simulink model "diff_controller_PID"  (R2024b)
settings: Solver=FixedStepAuto  StartTime=0.0  StopTime=inf  FixedStep=0.001  RelTol=1e-3  EnableMultiTasking=on
InitFcn:
  | Ts = 0.005;
  | diameter = 165; %mm
  | width = 441; %mm
libraries: arduinolib x4, simulink x2
settings Model: SimulationMode=external  ExtModeTrigDuration=2  Creator=System-10  LastModifiedBy=01149
settings SolverCC: AutoInsertRateTranBlk=on
settings OptimizationCC: EnhancedBackFolding=on  PassReuseOutputArgsAs=Individual arguments  ZeroExternalMemoryAtStartup=off  ZeroInternalMemoryAtStartup=off  MaxStackSize=64  OptimizeBlockOrder=speed  DifferentSizesBufferReuse=on  OptimizationCustomize=off  EfficientTunableParamExpr=on
settings DebuggingCC: ParameterTunabilityLossMsg=error
settings HardwareCC: ProdBitPerInt=16  ProdBitPerPointer=16  ProdBitPerSizeT=16  ProdBitPerPtrDiffT=16  ProdLargestAtomicFloat=None  ProdWordSize=8  ProdHWDeviceType=Atmel->AVR
settings SFSimCC: MATLABDynamicMemAlloc=off
settings RTWCC: Description=Embedded Coder  SystemTargetFile=ert.tlc  HardwareBoard=Arduino Mega 2560  TemplateMakefile=ert_default_tmf  GenerateReport=on  Toolchain=Arduino AVR  BuildConfiguration=Faster Runs  GPUComputeCapability=3.5
settings CodeAppCC: ForceParamTrailComments=on  IgnoreCustomStorageClasses=off  OperatorAnnotations=on  SimulinkDataObjDesc=on  SFDataObjDesc=on  InsertBlockDesc=on
settings ERTTargetCC: SupportContinuousTime=on  SupportVariableSizeSignals=on  ExtModeTransport=3  ExtModeStaticAlloc=on  ExtModeAutomaticAllocSize=off  ExtModeStaticAllocSize=2048  ExtModeMexFile=ext_xcp  ExtModeIntrfLevel=Level2 - Open  InlinedParameterPlacement=Hierarchical  DynamicArrayContainerType=coder::array

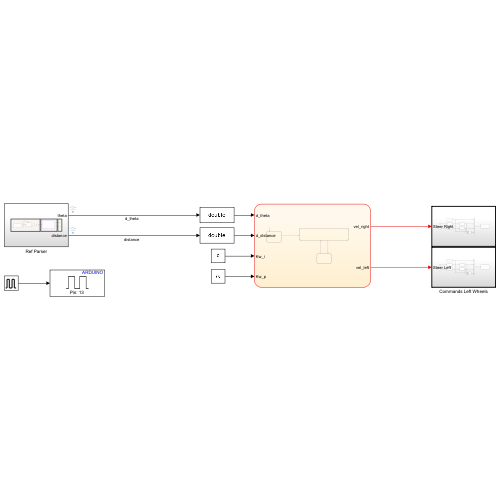
[thumbnail: Simulink's stored preview of the top-level diagram]
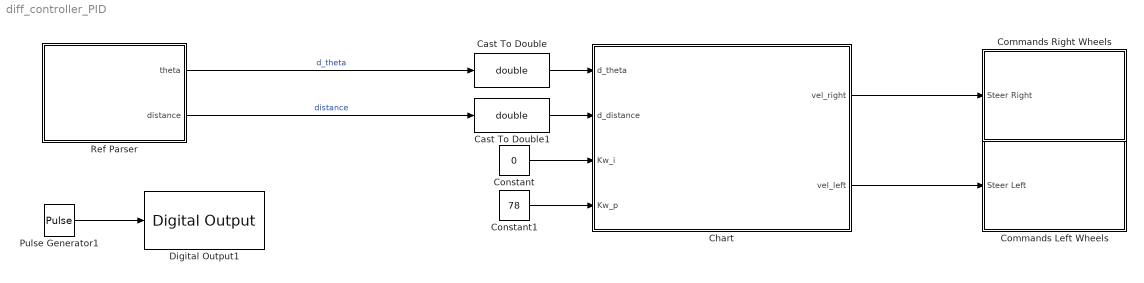
== system diff_controller_PID ==
  Cast To Double : DataTypeConversion  OutDataTypeStr=double  SaturateOnIntegerOverflow=off  RndMeth=Floor
  Cast To Double1 : DataTypeConversion  OutDataTypeStr=double  SaturateOnIntegerOverflow=off  RndMeth=Floor
  Chart : Stateflow chart  TreatAsAtomicUnit=on
  Commands Left Wheels : Subsystem  TreatAsAtomicUnit=on  SystemSampleTime=Ts
  Commands Right Wheels : Subsystem  TreatAsAtomicUnit=on  SystemSampleTime=Ts
  Constant : Constant  Value=0
  Constant1 : Constant  Value=78
  Digital Output1 : arduinolib/Digital Output  pinNumber=13  Direction=output  blockPlatform=arduino
  Pulse Generator1 : DiscretePulseGenerator  PulseType=Time based  PulseWidth=50
  Ref Parser : Subsystem
  wires:
  Pulse Generator1/1 -> Digital Output1/1
  Ref Parser/1(theta) -> Cast To Double/1  "d_theta"
  Ref Parser/2(distance) -> Cast To Double1/1  "distance"
  Constant/1 -> Chart/3(Kw_i)
  Constant1/1 -> Chart/4(Kw_p)
  Chart/1(vel_right) -> Commands Right Wheels/1(Steer Right)
  Chart/2(vel_left) -> Commands Left Wheels/1(Steer Left)
  Cast To Double/1 -> Chart/1(d_theta)
  Cast To Double1/1 -> Chart/2(d_distance)

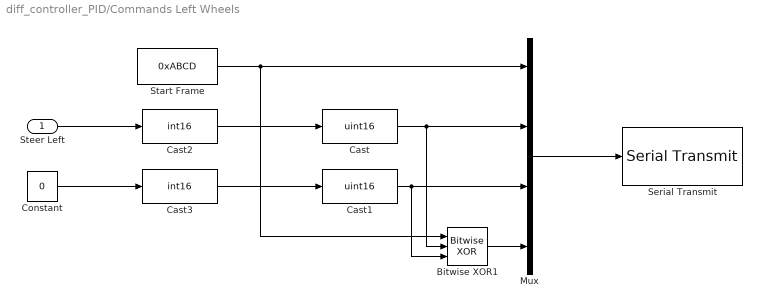
== system diff_controller_PID/Commands Left Wheels ==
  Steer Left : Inport
  Bitwise XOR1 : simulink/Logic and Bit Operations/Bitwise Operator  logicop=XOR  UseBitMask=off  NumInputPorts=3  BitMask=bin2dec('11011001')  BitMaskRealWorld=Stored Integer
      settings: LibrarySourceBlock=|
      | simulink/Quick Insert/Logic and Bit
      | Operations/Bitwise XOR
  Cast : DataTypeConversion  OutDataTypeStr=uint16  SaturateOnIntegerOverflow=off  RndMeth=Floor
  Cast1 : DataTypeConversion  OutDataTypeStr=uint16  SaturateOnIntegerOverflow=off  RndMeth=Floor
  Cast2 : DataTypeConversion  OutDataTypeStr=int16  SaturateOnIntegerOverflow=off  RndMeth=Floor
  Cast3 : DataTypeConversion  OutDataTypeStr=int16  SaturateOnIntegerOverflow=off  RndMeth=Floor
  Constant : Constant  Value=0
  Mux : Mux
  Serial Transmit : arduinolib/Serial Transmit  portNumber=3  sendmode=write  sendformat=Decimal  floatprecision=2  header=[]  terminator=[]  blockPlatform=arduino
  Start Frame : Constant  Value=0xABCD  OutDataTypeStr=uint16
  wires:
  Cast1/1 -> Bitwise XOR1/3, Mux/3
  Constant/1 -> Cast3/1
  Start Frame/1 -> Bitwise XOR1/1, Mux/1
  Mux/1 -> Serial Transmit/1
  Steer Left/1 -> Cast2/1
  Bitwise XOR1/1 -> Mux/4
  Cast/1 -> Bitwise XOR1/2, Mux/2
  Cast2/1 -> Cast/1
  Cast3/1 -> Cast1/1

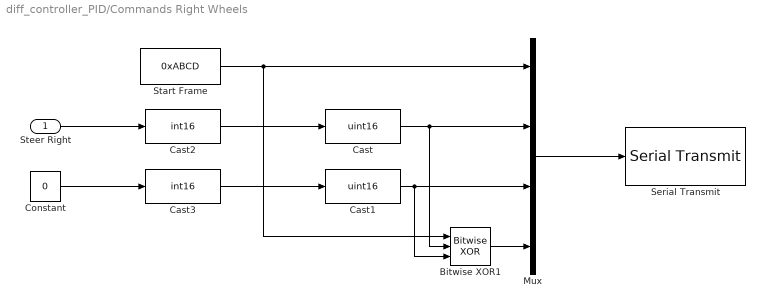
== system diff_controller_PID/Commands Right Wheels ==
  Steer Right : Inport
  Bitwise XOR1 : simulink/Logic and Bit Operations/Bitwise Operator  logicop=XOR  UseBitMask=off  NumInputPorts=3  BitMask=bin2dec('11011001')  BitMaskRealWorld=Stored Integer
      settings: LibrarySourceBlock=|
      | simulink/Quick Insert/Logic and Bit
      | Operations/Bitwise XOR
  Cast : DataTypeConversion  OutDataTypeStr=uint16  SaturateOnIntegerOverflow=off  RndMeth=Floor
  Cast1 : DataTypeConversion  OutDataTypeStr=uint16  SaturateOnIntegerOverflow=off  RndMeth=Floor
  Cast2 : DataTypeConversion  OutDataTypeStr=int16  SaturateOnIntegerOverflow=off  RndMeth=Floor
  Cast3 : DataTypeConversion  OutDataTypeStr=int16  SaturateOnIntegerOverflow=off  RndMeth=Floor
  Constant : Constant  Value=0
  Mux : Mux
  Serial Transmit : arduinolib/Serial Transmit  portNumber=2  sendmode=write  sendformat=Decimal  floatprecision=2  header=[]  terminator=[]  blockPlatform=arduino
  Start Frame : Constant  Value=0xABCD  OutDataTypeStr=uint16
  wires:
  Cast1/1 -> Bitwise XOR1/3, Mux/3
  Start Frame/1 -> Bitwise XOR1/1, Mux/1
  Mux/1 -> Serial Transmit/1
  Steer Right/1 -> Cast2/1
  Bitwise XOR1/1 -> Mux/4
  Cast/1 -> Bitwise XOR1/2, Mux/2
  Cast2/1 -> Cast/1
  Cast3/1 -> Cast1/1
  Constant/1 -> Cast3/1

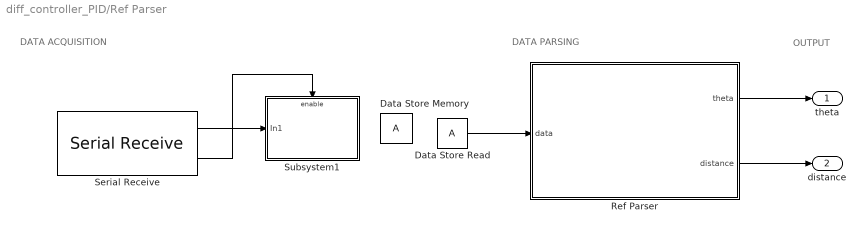
== system diff_controller_PID/Ref Parser ==
  note: DATA ACQUISITION
  note: DATA PARSING
  note: OUTPUT
  Data Store Memory : DataStoreMemory  WriteAfterWriteMsg=warning  InitialValue=88  ShowAdditionalParam=off  OutDataTypeStr=uint8  Dimensions=[1 24]
  Data Store Read : DataStoreRead  IndexOptions=Index vector (dialog)  Indices=1  OutputSizes=1
  Ref Parser : MATLAB Function  TreatAsAtomicUnit=on
  Serial Receive : arduinolib/Serial Receive  portNumber=1  DataType=uint8  blockPlatform=arduino  TimeOut=10  MaxDataLength=16  isARMArch=off  DataLengthOption=Length via dialog  Datalength=24  Header=[]  Terminator=[]  SampleTime=Ts  ShowOutStatus=on
  Subsystem1 : Subsystem
  theta : Outport
  distance : Outport  Port=2
  wires:
  Serial Receive/2 -> Subsystem1/Enable
  Data Store Read/1 -> Ref Parser/1(data)
  Serial Receive/1 -> Subsystem1/1(In1)
  Ref Parser/1(theta) -> theta/1
  Ref Parser/2(distance) -> distance/1

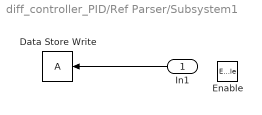
== system diff_controller_PID/Ref Parser/Subsystem1 ==
  In1 : Inport
  Enable : EnablePort
  Data Store Write : DataStoreWrite  IndexOptions=Index vector (dialog)  Indices=1  OutputSizes=1
  wires:
  In1/1 -> Data Store Write/1

== stateflow chart diff_controller_PID/Chart ==
  settings: updateMethod=DISCRETE  sampleTime=Ts
  state Moving
    during:
    d_theta_sum = d_theta_sum + d_theta;
    vel_left = -(vel_base + ((Kw_p*d_theta*1/pi) + Kw_i*d_theta_sum));
    vel_right = (vel_base - ((Kw_p*d_theta*1/pi) + Kw_i*d_theta_sum));
  state Init
    entry:
    vel_right = 0;
    vel_left = 0;
    d_theta_sum = 0;
  state Stopped
    entry:
    vel_right = 0;
    vel_left = 0;
    d_theta_sum = 0;
  (default) -> Init
  Init -> Moving : after(10,sec)
  Stopped -> Moving : [d_distance > 0.5 || d_distance < -0.5]
  Moving -> Stopped : [d_distance <= 0.5 && d_distance >= -0.5]
  data: vel_right output; vel_left output; d_theta input; d_distance input; vel_base local =200; d_theta_sum local =0; Kw_i input =0; Kw_p input =1

== matlab function diff_controller_PID/Ref Parser/Ref Parser ==
  settings: updateMethod=DISCRETE  sampleTime=Ts
  data: data input; theta output size=[1 1]; distance output size=[1 1]
function [theta, distance] = process_feedback(data)
    % process_feedback searches an array of uint8 values for a valid packet.
    %
    % Packet protocol:
    %   HEADER (uint8)        : 0xAA
    %   THETA (4 x uint8)     : desired theta in rad (stored as 4 bytes)
    %   DISTANCE (4 x uint8)  : desired distance in meter (stored as 4 bytes)
    %   Checksum (uint8)      : XOR checksum of HEADER, THETA, and DISTANCE bytes
    %   Dummy Byte (uint8)    : must equal 0xEE
    %   TERMINATOR (uint8)    : must equal 0xEF
    %
    % If a valid packet is found, the function decodes THETA and DISTANCE;
    % if none is found, it returns the last valid values.
    %
    % The packet is 12 bytes long.
    %

    persistent lastTheta lastDistance;
    if isempty(lastTheta)
        lastTheta = single(0);
    end
    if isempty(lastDistance)
        lastDistance = single(0);
    end

    HEADER   = uint8(170);  % 0xAA
    DUMMY    = uint8(238);  % 0xEE
    TERMINATOR = uint8(239); % 0xEF
    PACKET_SIZE = 12;       

    data = data(:)';

    for i = 1:(length(data) - PACKET_SIZE + 1)
        if data(i) == HEADER
            packet = data(i:(i+PACKET_SIZE-1));

            % Extract fields from the packet:
            % - Byte 1: HEADER (already checked)
            % - Bytes 2-5: THETA bytes
            % - Bytes 6-9: DISTANCE bytes
            % - Byte 10: Checksum
            % - Byte 11: Dummy byte (should equal 0xEE)
            % - Byte 12: Terminator (should equal 0xEF)
            thetaBytes    = packet(2:5);
            distanceBytes = packet(6:9);
            receivedChecksum = packet(10);
            dummy         = packet(11);
            terminator    = packet(12);

            if dummy ~= DUMMY || terminator ~= TERMINATOR
                continue; 
            end
            
            computedChecksum = packet(1);
            for j = 2:9
                computedChecksum = bitxor(computedChecksum, packet(j));
            end

            if computedChecksum ~= receivedChecksum
                continue; 
            end

            theta    = typecast(uint8(thetaBytes), 'single');
            distance = typecast(uint8(distanceBytes), 'single');

            lastTheta = theta;
            lastDistance = distance;
        end
    end

    theta    = lastTheta;
    distance = lastDistance;
   
end
